simulink model "discrete_vs_continuous"  (R2016a)
settings: Solver=VariableStepAuto  StartTime=0.0  StopTime=.1  RelTol=1e-3
values from neighbouring files (symbols this model uses):
  K = place(A,B,P)    [linearize.m]
  K_d = acker(A_d,B_d,P_d)    [linearize.m]
settings Model: Creator=manuel  LastModifiedBy=manuel

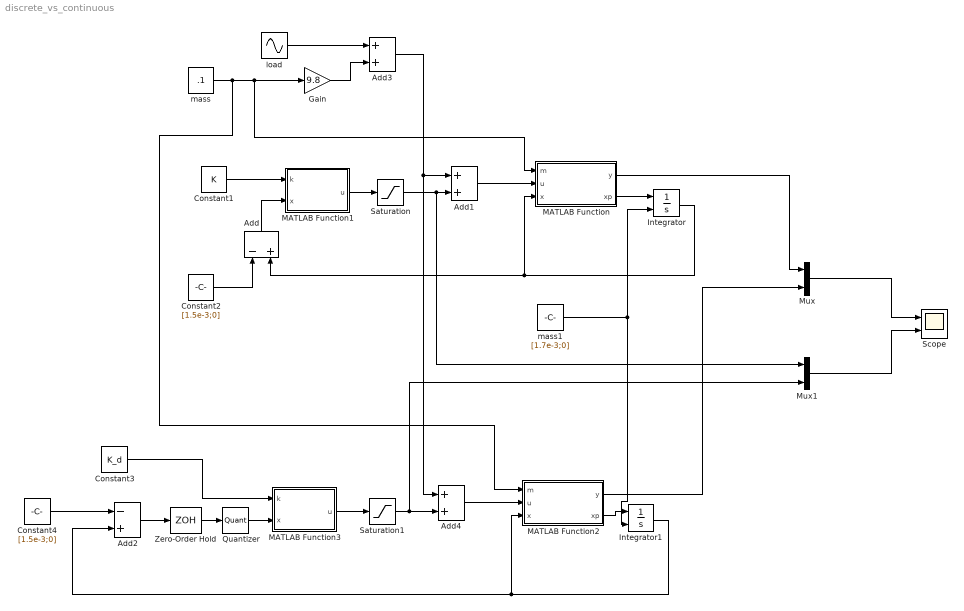
== system discrete_vs_continuous ==
  Add : Sum  Inputs=-+
  Add1 : Sum
  Add2 : Sum  Inputs=-+
  Add3 : Sum
  Add4 : Sum
  Constant1 : Constant  Value=K
  Constant2 : Constant  Value=[1.5e-3;0]
  Constant3 : Constant  Value=K_d
  Constant4 : Constant  Value=[1.5e-3;0]
  Gain : Gain  Gain=9.8
  Integrator : Integrator  InitialConditionSource=external  InitialCondition=[1.6e-3;0]  LimitOutput=on  UpperSaturationLimit=[2e-3;inf]  LowerSaturationLimit=[1e-3;-inf]
  Integrator1 : Integrator  InitialConditionSource=external  InitialCondition=[1.5e-3;0]  LimitOutput=on  UpperSaturationLimit=[2e-3;inf]  LowerSaturationLimit=[1e-3;-inf]
  MATLAB Function : MATLAB Function  TreatAsAtomicUnit=on
  MATLAB Function1 : MATLAB Function  TreatAsAtomicUnit=on
  MATLAB Function2 : MATLAB Function  TreatAsAtomicUnit=on
  MATLAB Function3 : MATLAB Function  TreatAsAtomicUnit=on
  Mux : Mux  Inputs=2
  Mux1 : Mux  Inputs=2
  Quantizer : Quantizer  QuantizationInterval=1e-4
  Saturation : Saturate  UpperLimit=9.8  LowerLimit=-9.8
  Saturation1 : Saturate  UpperLimit=9.8  LowerLimit=-9.8
  Scope : Scope  NumInputPorts=2
  Zero-Order Hold : ZeroOrderHold  SampleTime=1e-3
  load : Sin  Amplitude=2  Frequency=2*pi*100  SampleTime=0
  mass : Constant  Value=.1
  mass1 : Constant  Value=[1.7e-3;0]
  wires:
  MATLAB Function/2(xp) -> Integrator/1
  Integrator/1 -> MATLAB Function/3(x), Add/2
  MATLAB Function/1(y) -> Mux/1
  Constant1/1 -> MATLAB Function1/1(k)
  Constant2/1 -> Add/1
  Add/1 -> MATLAB Function1/2(x)
  Add1/1 -> MATLAB Function/2(u)
  Gain/1 -> Add3/2
  load/1 -> Add3/1
  MATLAB Function2/2(xp) -> Integrator1/1
  Integrator1/1 -> Add2/2, MATLAB Function2/3(x)
  Constant3/1 -> MATLAB Function3/1(k)
  Constant4/1 -> Add2/1
  Add4/1 -> MATLAB Function2/2(u)
  Add3/1 -> Add4/1, Add1/1
  Add2/1 -> Zero-Order Hold/1
  Mux/1 -> Scope/1
  Mux1/1 -> Scope/2
  MATLAB Function2/1(y) -> Mux/2
  mass/1 -> MATLAB Function2/1(m), Gain/1, MATLAB Function/1(m)
  mass1/1 -> Integrator/2, Integrator1/2
  Zero-Order Hold/1 -> Quantizer/1
  Quantizer/1 -> MATLAB Function3/2(x)
  MATLAB Function1/1(u) -> Saturation/1
  Saturation/1 -> Mux1/1, Add1/2
  Saturation1/1 -> Mux1/2, Add4/2
  MATLAB Function3/1(u) -> Saturation1/1

== matlab function discrete_vs_continuous/MATLAB Function1 ==
  data: k input; x input; u output
function u = fcn(k,x)
%#codegen

u = -k'*x;

== matlab function discrete_vs_continuous/MATLAB Function ==
  data: m input; u input; x input; y output; xp output
function [y,xp] = mass_model(m,u,x)
%#codegen
A = [0 1
     0 0];
B = [0;
     1/m];
C = [1 0];

xp = A*x + B*u;
y = C*x;

== matlab function discrete_vs_continuous/MATLAB Function2 ==
  data: m input; u input; x input; y output; xp output
function [y,xp] = mass_model(m,u,x)
%#codegen
A = [0 1
     0 0];
B = [0;
     1/m];
C = [1 0];

xp = A*x + B*u;
y = C*x;

== matlab function discrete_vs_continuous/MATLAB Function3 ==
  data: k input; x input; u output
function u = fcn(k,x)
%#codegen

u = -k'*x;
